simulink model "Logan"  (R2024b)
settings: Solver=ode4  StartTime=0  StopTime=inf  FixedStep=0.01  RelTol=1e-3
values from neighbouring files (symbols this model uses):
  AltPoint = 100000    [Logan_init.m]
  area_secao = 79.402*1.5    (= 119.103)    [Logan_init.m]
  b = 9    [Logan_init.m]
  c = 15.252    [Logan_init.m]
  cp = 1003    [Logan_init.m]
  E = 110e9    (= 110000000000)    [Logan_init.m]
  eta_comb = 0.95    [Logan_init.m]
  Fuel_Freeze = 0    [Logan_init.m]
  g = 9.80665    [Logan_init.m]
  gamma = 1.4    [Logan_init.m]
  GammaRef_deg = 0    [Logan_init.m]
  h1 = 0.5746    [Logan_init.m]
  h2 = 0.7752    [Logan_init.m]
  h3 = 0.1502    [Logan_init.m]
  hc = h1 + h2 + h3    (= 1.5)    [Logan_init.m]
  he = 2.6    [Logan_init.m]
  Inertia = [Ixx 0 -Ixz; 0 Iyy 0; -Ixz 0 Izz]    [Logan_init.m]
  L = 22.5    [Logan_init.m]
  L_inlet = 5.5    [Logan_init.m]
  La = 5    [Logan_init.m]
  LHV = 120 * 10^6    (= 120000000)    [Logan_init.m]
  Ln0 = 4.8    [Logan_init.m]
  MachPoint = 10    [Logan_init.m]
  Manual_Control = 0    [Logan_init.m]
  MW_air = 28.85    [Logan_init.m]
  MW_H2 = 2.00    (= 2)    [Logan_init.m]
  PA_EngineMode = 0    [Logan_init.m]
  PA_LatMode = 2    [Logan_init.m]
  PA_LongMode = 2    [Logan_init.m]
  PA_TECSEngineInput = 0    [Logan_init.m]
  PhiPoint = 0    [Logan_init.m]
  R = 287    [Logan_init.m]
  RefMass_kg = 31000    [Logan_init.m]
  S = 91.5    [Logan_init.m]
  tau1 = 3.1    [Logan_init.m]
  tau2 = 18.23    [Logan_init.m]
  TECS_ON = 0    [Logan_init.m]
  theta1 = 4    [Logan_init.m]
  theta2 = 6    [Logan_init.m]
  theta_n = 4    [Logan_init.m]
  ThetaPoint = 0    [Logan_init.m]
  Trimming = 0    [Logan_init.m]    (also in Logan_trim.m)
  w = 3.000    (= 3)    [Logan_init.m]
  Waypoint_idx = 1    [Logan_init.m]
  Waypoints = [ ... (first row only)    [Logan_init.m]
  x_a = 3.7    [Logan_init.m]
  x_inlet = 6    [Logan_init.m]
  x_n0 = 3    [Logan_init.m]
  xf_m = 0    [Logan_init.m]
  y_cg = 0    [Logan_init.m]
  z_a = 0.4    [Logan_init.m]
  z_cg = -0.996    [Logan_init.m]
  z_inlet = 0.7    [Logan_init.m]
  zf_m = 0    [Logan_init.m]
undefined symbols (not defined in the file or in its folder): Earth, Receive, Send, WGS84
libraries: simulink x4, spsFirstOrderFilterLib x4, aerolibactuator x3, aerolibfltsims x2, aerolibatmos2 x1, aerolibtransform2 x1, aerolibanimutils x1, dspswit3 x1, spsEdgeDetectorLib x1
(part 5 of 5)

== matlab function Logan/Propulsion/ScramjetEngine/calculate_T3_M3 ==
  data: T1 input; T3 output; M1 input; f input; M3 output
function [T3, M3] = calculate_T3_M3(T1, M1, f)
    % Parâmetros constantes
    gamma = 1.4;          % Índice adiabático
    cp = 1003;            % Calor específico do ar (J/kg·K)
    cp_H2 = 14300;        % Calor específico do H2 (J/kg·K)
    T_ign_H2 = 845;       % Temperatura de ignição do H2 (K)
    T_init_H2 = 290;      % Temperatura inicial do H2 (K)
    f_st = 0.028;         % Razão estequiométrica do hidrogênio
    
    % Cálculo de T3 (Temperatura de ignição)
    T3 = ((cp + f * cp_H2) * T_ign_H2 - f_st * cp_H2 * T_init_H2) / cp;

    % Cálculo de M3 (Número de Mach após ignição)
    M3 = sqrt(max(((1 + ((gamma - 1) / 2) * M1^2) * (T1 / T3) - 1) / ((gamma - 1) / 2),0));

end

== matlab function Logan/Propulsion/Engine Forces ==
  data: pn input; M1 input; Fx_inlet output; p1 input; theta1 input; alpha input; h3 input; Ln input; La input; p6 input; tau1 input; tau2 input; Ln0 input; Ldoor input; x_n0 input; Fz_inlet output; Minlet output; Fx_a output; Fz_a output; Ma output; Fzn output; Mn output; x_inlet input; z_inlet input; x_a input; z_a input
function [Fx_inlet, Fz_inlet, Minlet, Fx_a, Fz_a, Ma, Fzn, Mn] = calc_forcas_momentos_extended(pn, M1, p1, theta1, alpha, h3, Ln, La,p6, tau1, tau2, Ln0, Ldoor, x_n0, x_inlet,z_inlet, x_a, z_a)
% Função Simulink para calcular forças e momentos no inlet, aftbody e nacelle.

% Entradas:
% M1      - Número de Mach upstream
% p1      - Pressão upstream [Pa]
% theta1   - Ângulo de deflexão upstream (graus)
% alpha   - Ângulo de ataque (graus)
% hi      - Altura característica no inlet [m]
% Ln      - Comprimento do inlet [m]
% La      - Comprimento da seção do aftbody [m]
% p1   - Pressão ambiente [Pa]
% p6      - Pressão característica [Pa]
% tau2    - Ângulo de deflexão downstream (graus)
% L_inlet - Comprimento da entrada [m]
% h_i     - Altura do aftbody [m]
% pn      - Pressão aplicada na nacele [Pa]
% Ln0     - Comprimento nominal da nacele [m]
% Ldoor   - Comprimento da porta do cowl [m]
% x_n0    - Posição característica da nacele [m]

% Saídas:
% Fx_inlet - Força axial no inlet [N]
% Fz_inlet - Força vertical no inlet [N]
% Minlet   - Momento no inlet [Nm]
% Fx_a     - Força axial no aftbody [N]
% Fz_a     - Força vertical no aftbody [N]
% Ma       - Momento no aftbody [Nm]
% Fzn      - Força na nacele [N]
% Mn       - Momento na nacele [Nm]

% Constante
gamma = 1.4; % Razão de calores específicos para o ar

% Conversão dos ângulos para radianos
theta1_rad = deg2rad(theta1);
alpha_rad = deg2rad(alpha);
tau1_rad = deg2rad(tau1);
tau2_rad = deg2rad(tau2);


%% Cálculos no Inlet
% Força axial no inlet
Fx_inlet = gamma * M1^2 * p1 * (1 - cos(theta1_rad + alpha_rad)) * h3;

% Força vertical no inlet
Fz_inlet = gamma * M1^2 * p1 * sin(theta1_rad + alpha_rad) * h3;

% Momento no inlet
Minlet = z_inlet * Fx_inlet - x_inlet * Fz_inlet;

%% Cálculos no Aftbody
% Força axial no aftbody
Fx_a = p1 * La * log(p6 / p1) * ((p6 / p1) / ((p6 / p1) - 1)) * tan(tau2_rad + tau1_rad);

% Força vertical no aftbody
Fz_a = -p1 * La * log(p6 / p1) * ((p6 / p1) / ((p6 / p1) - 1));

% Momento no aftbody
Ma = z_a * Fx_a - x_a * Fz_a;

%% Cálculos na Nacele

% Força na nacele
Fzn = -pn * Ln;

% Momento na nacele
Mn = -Fzn * (x_n0 + 0.5 * (Ldoor - Ln0));

end

== matlab function Logan/Propulsion/Nacelle_pressure ==
  data: theta_n input; M1 input; pn output; p1 input; alpha_deg input
function pn = calcula_pn(theta_n, M1, p1,alpha_deg)
% Função MATLAB compatível com Simulink para calcular a pressão p_n
% Substitui flowprandtlmeyer por lookup_prandtlmeyer.
%
% Entradas:
% M1           - Número de Mach upstream
% p1           - Pressão upstream [Pa]
% beta_deg     - Ângulo de choque (beta) em graus
% alpha_deg - Ângulo de ataque (em graus)
%
% Saída:
% pn - Pressão calculada após o choque ou expansão [Pa]

% Constante
gamma = 1.4; % Razão de calores específicos para o ar
theta_nacelle = theta_n + alpha_deg;
% Converte o ângulo de choque para radianos
beta = deg2rad(lookup_beta(theta_nacelle, M1));

% Determina o tipo de fenômeno: Choque Oblíquo ou Expansão Prandtl-Meyer
if alpha_deg >= 0
    % Cálculo para Choque Oblíquo
    p2_p1 = 1 + (2 * gamma / (gamma + 1)) * (M1^2 * sin(beta)^2 - 1);
    pn = p2_p1 * p1; % Pressão após o choque
else
    % Cálculo para Expansão Prandtl-Meyer
    
    % Determina o ângulo nu1 para Mach upstream (M1)
    nu1 = lookup_prandtlmeyer(M1, 'mach_to_nu'); % Obter nu dado Mach

    % Ângulo nu2 considerando a expansão
    nu2 = nu1 + abs(alpha_deg); % Novo nu com ângulo de ataque negativo

    % Resolve o Mach downstream (M2) para o ângulo nu2
    M2 = lookup_prandtlmeyer(nu2, 'nu_to_mach'); % Obter Mach dado nu2

    % Relação de pressão isentrópica para expansão
    pn = p1 * (1 + (gamma - 1) / 2 * M1^2)^(gamma / (gamma - 1)) / ...
             (1 + (gamma - 1) / 2 * M2^2)^(gamma / (gamma - 1));
end
end


function result = lookup_prandtlmeyer(input_value, query_type)
    %% Função para interpolar valores entre Mach e Ângulo Prandtl-Meyer (nu)
    % Parâmetros:
    % - input_value: Valor de entrada (Mach ou nu)
    % - query_type: Tipo de consulta ('nu_to_mach' ou 'mach_to_nu')
    %
    % Saída:
    % - result: Resultado interpolado (Mach ou nu)
    
     % Valores de Mach (preencha com os valores reais posteriormente)
    Mach_values = [1.1	1.2	1.3	1.4	1.5	1.6	1.7	1.8	1.9	2	2.1	2.2	2.3	2.4	2.5	2.6	2.7	2.8	2.9	3	3.1	3.2	3.3	3.4	3.5	3.6	3.7	3.8	3.9	4	4.1	4.2	4.3	4.4	4.5	4.6	4.7	4.8	4.9	5	5.1	5.2	5.3	5.4	5.5	5.6	5.7	5.8	5.9	6	6.1	6.2	6.3	6.4	6.5	6.6	6.7	6.8	6.9	7	7.1	7.2	7.3	7.4	7.5	7.6	7.7	7.8	7.9	8	8.1	8.2	8.3	8.4	8.5	8.6	8.7	8.8	8.9	9	9.1	9.2	9.3	9.4	9.5	9.6	9.7	9.8	9.9	10	10.1	10.2	10.3	10.4	10.5	10.6	10.7	10.8	10.9	11	11.1	11.2	11.3	11.4	11.5	11.6	11.7	11.8	11.9	12	12.1	12.2	12.3	12.4	12.5	12.6	12.7	12.8	12.9	13	13.1	13.2	13.3	13.4	13.5	13.6	13.7	13.8	13.9	14	14.1	14.2	14.3	14.4	14.5	14.6	14.7	14.8	14.9	15];
    
    % Valores de Ângulo Prandtl-Meyer nu correspondentes (preencha com os valores reais)
    Nu_values = [1.336200924	3.558233358	6.170285886	8.987020318	11.90520883	14.86035366	17.80990982	20.72506425	23.58613467	26.37976081	29.0970813	31.73249557	34.28279408	36.74653115	39.12356383	41.41470778	43.62147769	45.74588996	47.79031199	49.75734674	51.64974438	53.47033468	55.22197561	56.90751449	58.52975896	60.09145559	61.59527452	63.04379875	64.43951705	65.7848198	67.08199684	68.33323714	69.54062968	70.70616525	71.83173895	72.91915326	73.97012132	74.98627054	75.96914627	76.92021551	77.84087066	78.73243319	79.59615721	80.43323295	81.24479016	82.03190129	82.79558459	83.53680709	84.25648735	84.95549818	85.63466911	86.2947888	86.93660734	87.56083828	88.16816076	88.7592213	89.33463568	89.89499055	90.44084506	90.97273233	91.49116087	91.99661591	92.4895606	92.97043725	93.43966839	93.89765781	94.34479154	94.7814388	95.20795282	95.62467171	96.03191919	96.43000532	96.81922722	97.19986967	97.57220575	97.93649742	98.29299601	98.64194282	98.98356951	99.31809865	99.64574408	99.96671134	100.2811981	100.5893944	100.8914832	101.1876406	101.478036	101.7628327	102.0421879	102.3162532	102.5851746	102.849093	103.1081442	103.3624594	103.6121649	103.857383	104.0982316	104.3348244	104.5672716	104.7956794	105.0201507	105.2407849	105.457678	105.670923	105.8806099	106.0868259	106.2896551	106.4891792	106.6854774	106.8786261	107.0686996	107.2557699	107.4399067	107.6211777	107.7996483	107.9753824	108.1484415	108.3188856	108.486773	108.6521599	108.8151014	108.9756506	109.1338593	109.2897779	109.443455	109.5949383	109.7442739	109.8915068	110.0366806	110.1798378	110.3210197	110.4602666	110.5976176	110.7331108	110.8667834	110.9986714	111.1288101	111.2572338	111.3839758	111.5090686];

    % Verificar o tipo de consulta
    if strcmp(query_type, 'nu_to_mach')
        % Interpolação: Obter Mach dado nu
        result = interp1(Nu_values, Mach_values, input_value, 'linear', 'extrap');
        
    else strcmp(query_type, 'mach_to_nu');
        % Interpolação: Obter nu dado Mach
        result = interp1(Mach_values, Nu_values, input_value, 'linear', 'extrap');
    end
end

function beta = lookup_beta(theta, Mach)
    % Definir os valores de theta e Mach correspondentes às linhas e colunas
    theta_values = [5 10 15 20 25 30 35 40];
    Mach_values = [1 1.5 2 2.5 3 3.5 4 4.5 5 5.5 6 6.5 7 7.5 8 8.5 9 9.5 10 10.5 11 11.5 12 12.5 13];
    
    % Definir a tabela de ângulos de beta com os dados fornecidos
    beta_table = [
        47.89, 34.3,  27.42, 23.13, 20.18, 18.02, 16.37, 15.07, 14.02, 13.16, 12.44, 11.82, 11.3,  10.85, 10.45, 10.1,  9.79,  9.52,  9.27,  9.05,  8.86,  8.68,  8.51,  8.36,  8.23;
        56.68, 39.31, 31.85, 27.38, 24.38, 22.23, 20.62, 19.38, 18.39, 17.59, 16.93, 16.38, 15.92, 15.53, 15.19, 14.9,  14.65, 14.43, 14.23, 14.06, 13.91, 13.77, 13.65, 13.54, 13.44;
        45.34, 36.94, 32.24, 29.19, 27.06, 25.5,  24.32, 23.4,  22.67, 22.08, 21.6,  21.2,  20.86, 20.58, 20.33, 20.12, 19.94, 19.78, 19.64, 19.52, 19.41, 19.32, 19.23, 19.15, 19;
        53.42, 42.89, 37.76, 34.6,  32.46, 30.94, 29.8,  28.93, 28.26, 27.71, 27.28, 26.92, 26.62, 26.37, 26.16, 25.97, 25.82, 25.68, 25.56, 25.46, 25.37, 25.29, 25.21, 25.15, 25.09;
        50.25, 44.14, 40.69, 38.46, 36.91, 35.78, 34.93, 34.28, 33.76, 33.35, 33.01, 32.73, 32.5,  32.3,  32.14, 31.99, 31.87, 31.76, 31.67, 31.59, 31.51, 31.45, 31.39, 31.34, 31.29;
        52.01, 47.76, 45.22, 43.54, 42.34, 41.46, 40.79, 40.27, 39.85, 39.52, 39.24, 39.01, 38.82, 38.66, 38.52, 38.4,  38.29, 38.2,  38.12, 38.05, 37.99, 37.93, 37.88, 37.84, 37.8;
        57.19, 53.46, 51.3,  49.85, 48.83, 48.07, 47.48, 47.02, 46.65, 46.35, 46.11, 45.9,  45.73, 45.58, 45.45, 45.34, 45.24, 45.16, 45.08, 45.02, 44.96, 44.9,  44.86, 44.81, 44.78;
        64.34, 60.26, 58.4,  57.19, 56.32, 55.67, 55.17, 54.77, 54.44, 54.17, 53.95, 53.76, 53.6,  53.46, 53.34, 53.23, 53.14, 53.06, 52.98, 52.92, 52.86, 52.81, 52.76, 52.72, 52.68;
    ];

    % Interpolar ou extrapolar ao longo da dimensão Mach para cada valor de theta
    beta_theta = interp1(Mach_values, beta_table', Mach, 'linear', 'extrap');
    
    % Interpolar ou extrapolar ao longo da dimensão theta
    beta = interp1(theta_values, beta_theta, theta, 'linear', 'extrap');
end

== matlab function Logan/Propulsion/ScramjetEngine/calculate_shock_and_door ==
  data: theta1 input; ShockPoint output; Mach input; L_inlet input; hc input; door_length output
function [ShockPoint, door_length] = calculate_shock_and_door(theta1, Mach, L_inlet, hc)
% Função para calcular o ponto de choque horizontal e comprimento da porta
% Entradas:
% theta1          - Inclinação local da superfície (em graus)
% alpha           - Ângulo de ataque global (em graus)
% Mach            - Número de Mach
% hc              - Altura vertical do ponto de choque
% L1              - Comprimento total da porta
% distance_zero   - Deslocamento inicial (zero) da porta

% Saídas:
% ShockPoint      - Distância horizontal do ponto de choque
% door_length     - Comprimento efetivo da porta

% Ângulo global da superfície
theta1_global = theta1;

% Busca do ângulo de onda de choque beta1
beta1 = lookup_beta(theta1_global, Mach);

% Ângulo efetivo em radianos
beta_effective_rad = deg2rad(beta1 + theta1_global);

% Ponto de choque horizontal
ShockPoint = hc / tan(beta_effective_rad);

% Comprimento efetivo da porta
door_length = L_inlet - ShockPoint;
end


function beta = lookup_beta(theta, Mach)
    % Definir os valores de theta e Mach correspondentes às linhas e colunas
    theta_values = [5 10 15 20 25 30 35 40];
    Mach_values = [1 1.5 2 2.5 3 3.5 4 4.5 5 5.5 6 6.5 7 7.5 8 8.5 9 9.5 10 10.5 11 11.5 12 12.5 13];
    
    % Definir a tabela de ângulos de beta com os dados fornecidos
    beta_table = [
        47.89, 34.3,  27.42, 23.13, 20.18, 18.02, 16.37, 15.07, 14.02, 13.16, 12.44, 11.82, 11.3,  10.85, 10.45, 10.1,  9.79,  9.52,  9.27,  9.05,  8.86,  8.68,  8.51,  8.36,  8.23;
        56.68, 39.31, 31.85, 27.38, 24.38, 22.23, 20.62, 19.38, 18.39, 17.59, 16.93, 16.38, 15.92, 15.53, 15.19, 14.9,  14.65, 14.43, 14.23, 14.06, 13.91, 13.77, 13.65, 13.54, 13.44;
        45.34, 36.94, 32.24, 29.19, 27.06, 25.5,  24.32, 23.4,  22.67, 22.08, 21.6,  21.2,  20.86, 20.58, 20.33, 20.12, 19.94, 19.78, 19.64, 19.52, 19.41, 19.32, 19.23, 19.15, 19;
        53.42, 42.89, 37.76, 34.6,  32.46, 30.94, 29.8,  28.93, 28.26, 27.71, 27.28, 26.92, 26.62, 26.37, 26.16, 25.97, 25.82, 25.68, 25.56, 25.46, 25.37, 25.29, 25.21, 25.15, 25.09;
        50.25, 44.14, 40.69, 38.46, 36.91, 35.78, 34.93, 34.28, 33.76, 33.35, 33.01, 32.73, 32.5,  32.3,  32.14, 31.99, 31.87, 31.76, 31.67, 31.59, 31.51, 31.45, 31.39, 31.34, 31.29;
        52.01, 47.76, 45.22, 43.54, 42.34, 41.46, 40.79, 40.27, 39.85, 39.52, 39.24, 39.01, 38.82, 38.66, 38.52, 38.4,  38.29, 38.2,  38.12, 38.05, 37.99, 37.93, 37.88, 37.84, 37.8;
        57.19, 53.46, 51.3,  49.85, 48.83, 48.07, 47.48, 47.02, 46.65, 46.35, 46.11, 45.9,  45.73, 45.58, 45.45, 45.34, 45.24, 45.16, 45.08, 45.02, 44.96, 44.9,  44.86, 44.81, 44.78;
        64.34, 60.26, 58.4,  57.19, 56.32, 55.67, 55.17, 54.77, 54.44, 54.17, 53.95, 53.76, 53.6,  53.46, 53.34, 53.23, 53.14, 53.06, 52.98, 52.92, 52.86, 52.81, 52.76, 52.72, 52.68;
    ];

    % Interpolar ou extrapolar ao longo da dimensão Mach para cada valor de theta
    beta_theta = interp1(Mach_values, beta_table', Mach, 'linear', 'extrap');
    
    % Interpolar ou extrapolar ao longo da dimensão theta
    beta = interp1(theta_values, beta_theta, theta, 'linear', 'extrap');
end
